simulink model "Toast"  (R2021a)
settings: Solver=ode1  StartTime=0.0  StopTime=100  FixedStep=0.001  RelTol=1e-3
libraries: qbmove_library x3, eePwmGenerator x1, QB_pacer_lib x1, dspsrcs4 x1
settings Model: Creator=Marina Gnocco  LastModifiedBy=mgnocco

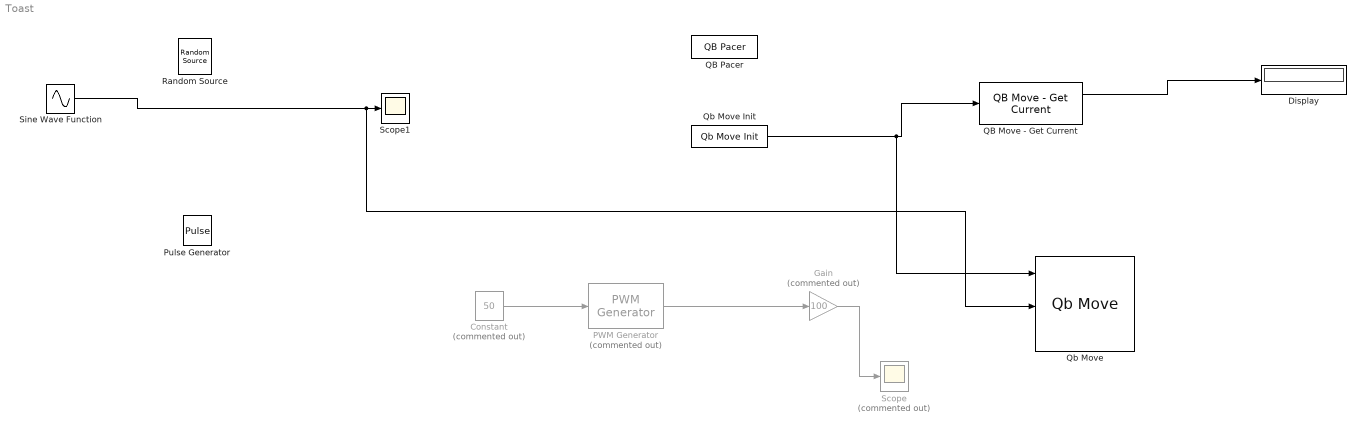
== system Toast ==
  Constant : Constant  Commented=on  Value=50
  Display : Display
  Gain : Gain  Commented=on  Gain=100
  PWM Generator : eePwmGenerator/PWM Generator  Commented=on  CarrCount=Up  Tper=1  Ts=0.1
  Pulse Generator : DiscretePulseGenerator  PulseType=Time based  Amplitude=100  Period=1  PulseWidth=50
  QB Move - Get Current : qbmove_library/QB Move - Get Current  ID=1  CONTROL_MODE=Prime Movers Positions  DAISY_CHAINING=off
      settings: SourceProductName=Qb Move Library
  QB Pacer : QB_pacer_lib/QB Pacer  simTimePerRealTime=1
      settings: SourceProductName=QB Pacer
  Qb Move : qbmove_library/Qb Move  ID=1  ACTIVE_COMM_DIRECTIONS=Both  CONTROL_MODE=Prime Movers Positions  DAISY_CHAINING=off  MAX_ANG=0  SW_LIMIT=inf  OFFSET=0  ACTIVATE=on  WDT=0.0  UNIT=TICK
      settings: SourceProductName=Qb Move Library
  Qb Move Init : qbmove_library/Qb Move Init  NUMBER_OF_COM='COM26'  BAUD_RATE_COM=2000000
      settings: SourceProductName=Qb Move Library
  Random Source : dspsrcs4/Random Source  SrcType=Uniform  NormMethod=Ziggurat  CltLength=12  MinVal=0  MaxVal=100  MeanVal=0  VarVal=1  RepMode=Not repeatable  rawSeed=1  IsInherit=off  SampMode=Continuous  SampTime=1  SampFrame=1  DataType=Double  OutComplex=Real  OutputFrames=off
  Scope : Scope  Commented=on
  Scope1 : Scope
  Sine Wave Function : Sin  Amplitude=50  Bias=50  SampleTime=0
  wires:
  Qb Move Init/1 -> Qb Move/1, QB Move - Get Current/1
  QB Move - Get Current/1 -> Display/1
  PWM Generator/1 -> Gain/1
  Constant/1 -> PWM Generator/1
  Gain/1 -> Scope/1
  Sine Wave Function/1 -> Qb Move/2, Scope1/1
